simulink model "simulink_template_1_1"  (R2024b)
settings: Solver=VariableStepAuto  StartTime=0.0  StopTime=T_SIMULATION  RelTol=1e-3
values from neighbouring files (symbols this model uses):
  d = 0.165    [script_1_1.m]
  OMEGA_L = 1    [script_1_1.m]
  OMEGA_R = 1    [script_1_1.m]
  Q_INITIAL = [0;0;0]    [script_1_1.m]
  r = 0.03    [script_1_1.m]
settings Model: Creator=alber  LastModifiedBy=eugen

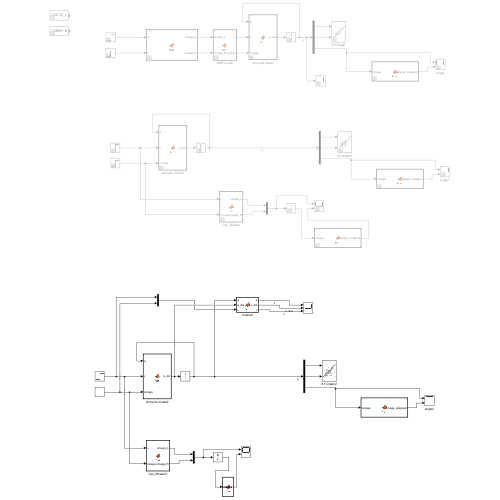
[thumbnail: Simulink's stored preview of the top-level diagram]
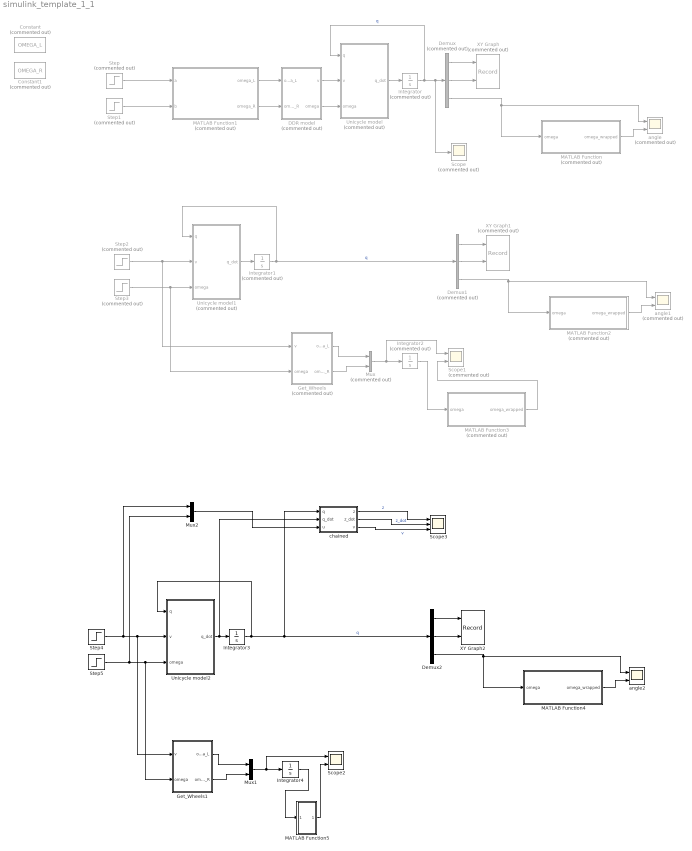
== system simulink_template_1_1 ==
  Constant : Constant  Commented=on  Value=OMEGA_L
  Constant1 : Constant  Commented=on  Value=OMEGA_R
  DDR model : MATLAB Function  Commented=on  TreatAsAtomicUnit=on
  Demux : Demux  Commented=on  Outputs=3
  Demux1 : Demux  Commented=on  Outputs=3
  Demux2 : Demux  Outputs=3
  Get_Wheels : MATLAB Function  Commented=on  TreatAsAtomicUnit=on
  Get_Wheels1 : MATLAB Function  TreatAsAtomicUnit=on
  Integrator : Integrator  Commented=on  InitialCondition=Q_INITIAL
  Integrator1 : Integrator  Commented=on  InitialCondition=Q_INITIAL
  Integrator2 : Integrator  Commented=on
  Integrator3 : Integrator  InitialCondition=Q_INITIAL
  Integrator4 : Integrator
  MATLAB Function : MATLAB Function  Commented=on  TreatAsAtomicUnit=on
  MATLAB Function1 : MATLAB Function  Commented=on  TreatAsAtomicUnit=on
  MATLAB Function2 : MATLAB Function  Commented=on  TreatAsAtomicUnit=on
  MATLAB Function3 : MATLAB Function  Commented=on  TreatAsAtomicUnit=on
  MATLAB Function4 : MATLAB Function  TreatAsAtomicUnit=on
  MATLAB Function5 : MATLAB Function  TreatAsAtomicUnit=on
  Mux : Mux  Commented=on  Inputs=2
  Mux1 : Mux  Inputs=2
  Mux2 : Mux  Inputs=2
  Scope : Scope  Commented=on
  Scope1 : Scope  Commented=on  NumInputPorts=2
  Scope2 : Scope  NumInputPorts=2
  Scope3 : Scope  NumInputPorts=3
  Step : Step  Commented=on  SampleTime=0
  Step1 : Step  Commented=on  After=20  SampleTime=0
  Step2 : Step  Commented=on  After=2  SampleTime=0
  Step3 : Step  Commented=on  After=1.5  SampleTime=0
  Step4 : Step  After=2  SampleTime=0
  Step5 : Step  After=1.5  SampleTime=0
  Unicycle model : MATLAB Function  Commented=on  TreatAsAtomicUnit=on
  Unicycle model1 : MATLAB Function  Commented=on  TreatAsAtomicUnit=on
  Unicycle model2 : MATLAB Function  TreatAsAtomicUnit=on
  XY Graph : Record  Commented=on  FileSettingsInternal="{\"entries\":[{\"content\":{\"excelSettings\":{\"content\":{},\"type\":\"Streamout.ExcelSettings\"}},\"type\":\"Streamout.FileSettingStorage\",\"uuid\":\"\"}],\"packageUris\":[\"http:\\/\\/schema.mathworks.com\\/mf0\\/streamout_blocks\\/R2020a\"],\"version\":\"1.0\"}"  Layout=[1 1]  SignalsInternal="{\"entries\":[{\"content\":{},\"type\":\"RecordBlkView.InputSignals\",\"uuid\":\"\"}],\"packageUris\":[\"http:\\/\\/schema.mathworks.com\\/mf0\\/streamout_blocks\\/R2020a\"],\"version\":\"1.0\"}"  VisualizationBindings="{\"xyplotplugin\":{\"info\":[{\"series\":[],\"subplotID\":1}]}}"  CompatibilityTag=XY
  XY Graph1 : Record  Commented=on  FileSettingsInternal="{\"entries\":[{\"content\":{\"excelSettings\":{\"content\":{},\"type\":\"Streamout.ExcelSettings\"}},\"type\":\"Streamout.FileSettingStorage\",\"uuid\":\"\"}],\"packageUris\":[\"http:\\/\\/schema.mathworks.com\\/mf0\\/streamout_blocks\\/R2020a\"],\"version\":\"1.0\"}"  Layout=[1 1]  SignalsInternal="{\"entries\":[{\"content\":{},\"type\":\"RecordBlkView.InputSignals\",\"uuid\":\"\"}],\"packageUris\":[\"http:\\/\\/schema.mathworks.com\\/mf0\\/streamout_blocks\\/R2020a\"],\"version\":\"1.0\"}"  VisualizationBindings="{\"xyplotplugin\":{\"info\":[{\"series\":[],\"subplotID\":1}]}}"  CompatibilityTag=XY
  XY Graph2 : Record  FileSettingsInternal="{\"entries\":[{\"content\":{\"excelSettings\":{\"content\":{},\"type\":\"Streamout.ExcelSettings\"}},\"type\":\"Streamout.FileSettingStorage\",\"uuid\":\"\"}],\"packageUris\":[\"http:\\/\\/schema.mathworks.com\\/mf0\\/streamout_blocks\\/R2020a\"],\"version\":\"1.0\"}"  Layout=[1 1]  SignalsInternal="{\"entries\":[{\"content\":{\"signals\":[{\"content\":{\"blockPath\":[],\"dimensions\":[1,1],\"domain\":\"\",\"lineColor\":\"#a2142f\",\"plots\":[ 1 ],\"port\":1,\"sid\":[\"\"],\"signalID\":1,\"signalName\":\"Demux2:1\"},\"type\":\"RecordBlkView.Signal\",\"uuid\":\"\"},{\"content\":{\"blockPath\":[],\"dimensions\":[1,1],\"domain\":\"\",\"lineColor\":\"#139fff\",\"plots\":[ 1 ],\"port\":2,\"sid\":[\"\"],\"signalID\":2,\"signalName\":\"Demux2:2\"},\"type\":\"RecordBlkView.Signal\",\"uuid\":\"\"}]},\"type\":\"RecordBlkView.InputSignals\",\"uuid\":\"\"}],\"packageUris\":[\"http:\\/\\/schema.mathworks.com\\/mf0\\/streamout_blocks\\/R2020a\"],\"version\":\"1.0\"}"  VisualizationBindings="{\"xyplotplugin\":{\"info\":[{\"series\":[{\"bindingParametersList\":[{\"parameter\":\"X-Axis\",\"signalID\":1,\"signalName\":\"Demux2:1\"},{\"parameter\":\"Y-Axis\",\"signalID\":2,\"signalName\":\"Demux2:2\"}],\"seriesID\":0}],\"subplotID\":1}]}}"  CompatibilityTag=XY
  angle : Scope  Commented=on  NumInputPorts=2
  angle1 : Scope  Commented=on  NumInputPorts=2
  angle2 : Scope  NumInputPorts=2
  chained : MATLAB Function  TreatAsAtomicUnit=on
  wires:
  Unicycle model/1(q_dot) -> Integrator/1
  DDR model/2(omega) -> Unicycle model/3(omega)
  DDR model/1(v) -> Unicycle model/2(v)
  Integrator/1 -> Scope/1, Demux/1, Unicycle model/1(q)  "q"
  Demux/2 -> XY Graph/2
  Demux/1 -> XY Graph/1
  MATLAB Function1/2(omega_R) -> DDR model/2(omega_R)
  MATLAB Function1/1(omega_L) -> DDR model/1(omega_L)
  Step/1 -> MATLAB Function1/1(a)
  Step1/1 -> MATLAB Function1/2(b)
  MATLAB Function/1(omega_wrapped) -> angle/2
  Demux/3 -> angle/1, MATLAB Function/1(omega)
  Demux1/3 -> angle1/1, MATLAB Function2/1(omega)
  Demux1/1 -> XY Graph1/1
  MATLAB Function2/1(omega_wrapped) -> angle1/2
  Integrator1/1 -> Demux1/1, Unicycle model1/1(q)  "q"
  Unicycle model1/1(q_dot) -> Integrator1/1
  Demux1/2 -> XY Graph1/2
  Step2/1 -> Get_Wheels/1(v), Unicycle model1/2(v)
  Step3/1 -> Get_Wheels/2(omega), Unicycle model1/3(omega)
  Get_Wheels/1(omega_L) -> Mux/1
  Get_Wheels/2(omega_R) -> Mux/2
  Integrator2/1 -> MATLAB Function3/1(omega)
  Mux/1 -> Scope1/1, Integrator2/1
  MATLAB Function3/1(omega_wrapped) -> Scope1/2
  Get_Wheels1/2(omega_R) -> Mux1/2
  Get_Wheels1/1(omega_L) -> Mux1/1
  Mux1/1 -> Scope2/1, Integrator4/1
  MATLAB Function5/1(omega_wrapped) -> Scope2/2
  Step5/1 -> Mux2/2, Get_Wheels1/2(omega), Unicycle model2/3(omega)
  Demux2/2 -> XY Graph2/2
  Unicycle model2/1(q_dot) -> chained/2(q_dot), Integrator3/1
  Step4/1 -> Mux2/1, Get_Wheels1/1(v), Unicycle model2/2(v)
  Integrator4/1 -> MATLAB Function5/1(omega)
  Integrator3/1 -> chained/1(q), Demux2/1, Unicycle model2/1(q)  "q"
  Demux2/3 -> angle2/1, MATLAB Function4/1(omega)
  Demux2/1 -> XY Graph2/1
  MATLAB Function4/1(omega_wrapped) -> angle2/2
  Mux2/1 -> chained/3(u)
  chained/1(z) -> Scope3/1  "z"
  chained/2(z_dot) -> Scope3/2  "z_dot"
  chained/3(v) -> Scope3/3  "v"

== matlab function simulink_template_1_1/MATLAB Function5 ==
  data: omega input; omega_wrapped output
function omega_wrapped = fcn(omega)

omega_wrapped = wrapToPi(omega);

== matlab function simulink_template_1_1/Unicycle model2 ==
  data: q input; v input; q_dot output; omega input; r parameter; d parameter
function q_dot = fcn(q, v, omega, r, d)
%write the unicycle model
%q_dot= zeros(3,1);
q_dot = [cos(q(3))*v; sin(q(3))*v; omega];

== matlab function simulink_template_1_1/Unicycle model ==
  data: q input; v input; q_dot output; omega input; r parameter; d parameter
function q_dot = fcn(q, v, omega, r, d)
%write the unicycle model
%q_dot= zeros(3,1);
q_dot = [cos(q(3))*v; sin(q(3))*v; omega];

== matlab function simulink_template_1_1/chained ==
  data: q input; q_dot input; u input; z output; z_dot output; v output
function [z,z_dot,v]= fcn(q,q_dot,u)

z = [q(3);
    q(1)*cos(q(3)) + q(2)*sin(q(3));
    q(1)*sin(q(3)) - q(2)*cos(q(3));
    ];

v = [u(2);u(1)-z(3)*u(2)];

z_dot= [v(1);v(2);z(2)*v(1)];

== matlab function simulink_template_1_1/DDR model ==
  data: omega_L input; v output; omega_R input; omega output; r parameter; d parameter
function [v, omega] = fcn(omega_L, omega_R, r, d)
%write the DDR model and return v and omega
v     = (r*omega_L + r*omega_R) / 2;
omega = (-r*omega_L + r*omega_R) / d;

== matlab function simulink_template_1_1/MATLAB Function ==
  data: omega input; omega_wrapped output
function omega_wrapped = fcn(omega)

omega_wrapped = wrapToPi(omega);

== matlab function simulink_template_1_1/MATLAB Function1 ==
  data: a input; omega_L output; b input; omega_R output
function [omega_L, omega_R]= fcn(a,b)

omega_L = a;
omega_R = b;

== matlab function simulink_template_1_1/Get_Wheels ==
  data: v input; omega_L output; omega input; omega_R output; d parameter
function [omega_L, omega_R] = fcn(v, omega, d)
%write the DDR model and return v and omega

omega_L = (v - d*omega) / 2;
omega_R = (v + d*omega) / 2;

== matlab function simulink_template_1_1/MATLAB Function2 ==
  data: omega input; omega_wrapped output
function omega_wrapped = fcn(omega)

omega_wrapped = wrapToPi(omega);

== matlab function simulink_template_1_1/MATLAB Function3 ==
  data: omega input; omega_wrapped output
function omega_wrapped = fcn(omega)

omega_wrapped = wrapToPi(omega);

== matlab function simulink_template_1_1/Unicycle model1 ==
  data: q input; v input; q_dot output; omega input; r parameter; d parameter
function q_dot = fcn(q, v, omega, r, d)
%write the unicycle model
%q_dot= zeros(3,1);
q_dot = [cos(q(3))*v; sin(q(3))*v; omega];

== matlab function simulink_template_1_1/Get_Wheels1 ==
  data: v input; omega_L output; omega input; omega_R output; d parameter
function [omega_L, omega_R] = fcn(v, omega, d)
%write the DDR model and return v and omega

omega_L = (v - d*omega) / 2;
omega_R = (v + d*omega) / 2;

== matlab function simulink_template_1_1/MATLAB Function4 ==
  data: omega input; omega_wrapped output
function omega_wrapped = fcn(omega)

omega_wrapped = wrapToPi(omega);
